simulink model "Luenb_no_integr_sim_model"  (R2020a)
settings: Solver=ode3  StartTime=0.0  StopTime=600  FixedStep=Ts  RelTol=1e-3  EnableMultiTasking=on
values from neighbouring files (symbols this model uses):
  A = Model.A    [GPB1_estimation.m]    (also in GPB1_estimation_BT.m; GPB2_estimation.m)
  B = Model.B    [GPB1_estimation_BT.m]
  C = Model.C    [GPB1_estimation.m]    (also in GPB1_estimation_BT.m; GPB2_estimation.m; MKFObserverA.m = obj.filters{f}.C)
  K = Pred_P * C{j}' / S    [GPB1_estimation.m]    (also in GPB1_estimation_BT.m; GPB2_estimation.m)
  x0 = zeros(n, 1)    [AbstractLinearFilter.m]    (also in KalmanFilter.m; KalmanFilterSS_sfunc.m = obs.xkp1_est; MEKF_observer_RODD.m; MKFObserver.m)
undefined symbols (not defined in the file or in its folder): Ts
settings Model: Creator=desbiens  LastModifiedBy=billtubbs
settings DataIOCC: LimitDataPoints=on  SaveFormat=Array  SignalLoggingSaveFormat=ModelDataLogs  ReturnWorkspaceOutputs=off
settings OptimizationCC: ExpressionDepthLimit=2147483647  InitFltsAndDblsToZero=on  LifeSpan=inf
settings DebuggingCC: UnderspecifiedInitializationDetection=Classic  MergeDetectMultiDrivingBlocksExec=none  SolverPrmCheckMsg=warning  FcnCallInpInsideContextMsg=warning  StateNameClashWarn=warning  SFUnexpectedBacktrackingDiag=warning  SFNoUnconditionalDefaultTransitionDiag=warning  SFExecutionAtInitializationDiag=none  ArithmeticOperatorsInVariantConditions=warning
settings HardwareCC: ProdBitPerPointer=32  ProdBitPerSizeT=32  ProdBitPerPtrDiffT=32  ProdLargestAtomicFloat=None  ProdIntDivRoundTo=Undefined  ProdEndianess=Unspecified  ProdWordSize=32  ProdHWDeviceType=32-bit Generic
settings ModelReferenceCC: PropagateSignalLabelsOutOfModel=off
settings SFSimCC: SimUseLocalCustomCode=off  CustomCodeUndefinedFunction=UseInterfaceOnly
settings RTWCC: RTWUseLocalCustomCode=off
settings CodeAppCC: StateflowObjectComments=on
settings GRTTargetCC: TargetLangStandard=C89/C90 (ANSI)  CombineOutputUpdateFcns=off  GRTInterface=on
settings ConfigComp: CovMetricSettings=dw  CovHtmlReporting=on  CovSaveCumulativeToWorkspaceVar=on  CovSaveSingleToWorkspaceVar=on  CovExternalEMLEnable=off

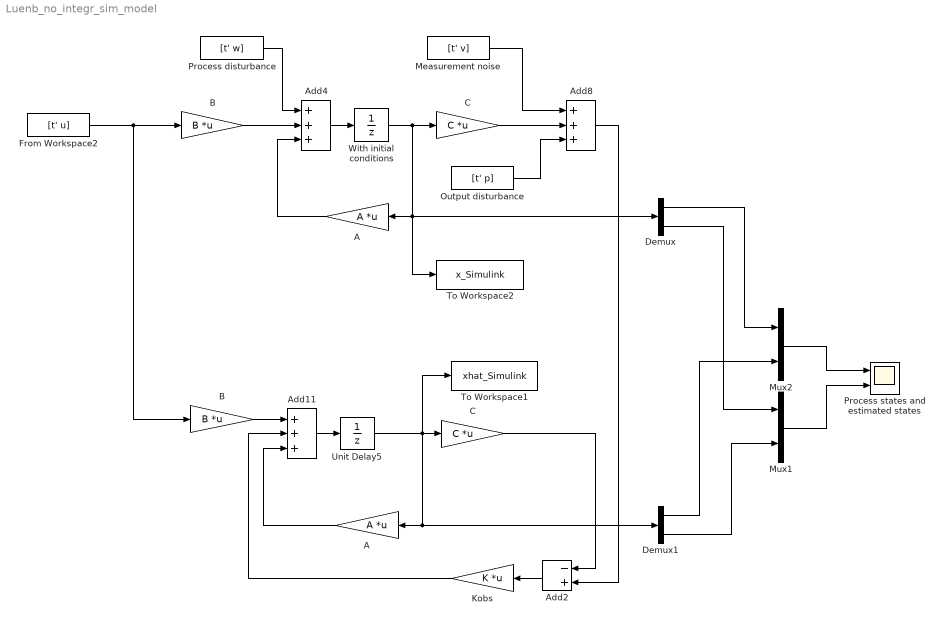
== system Luenb_no_integr_sim_model ==
  A : Gain  Gain=A  Multiplication=Matrix(K*u)
  "A " : Gain  Gain=A  Multiplication=Matrix(K*u)
  Add11 : Sum  Inputs=+++
  Add2 : Sum  Inputs=-+
  Add4 : Sum  Inputs=+++
  Add8 : Sum  Inputs=+++
  B : Gain  Gain=B  Multiplication=Matrix(K*u)
  "B " : Gain  Gain=B  Multiplication=Matrix(K*u)
  C : Gain  Gain=C  Multiplication=Matrix(K*u)
  "C " : Gain  Gain=C  Multiplication=Matrix(K*u)
  Demux : Demux  Outputs=2
  Demux1 : Demux  Outputs=2
  From Workspace2 : FromWorkspace  VariableName=[t' u]
  Kobs : Gain  Gain=K  Multiplication=Matrix(K*u)
  Measurement noise : FromWorkspace  VariableName=[t' v]
  Mux1 : Mux  Inputs=2
  Mux2 : Mux  Inputs=2
  Output disturbance : FromWorkspace  VariableName=[t' p]
  Process disturbance : FromWorkspace  VariableName=[t' w]
  Process states and estimated states : Scope  NumInputPorts=2
  To Workspace1 : ToWorkspace  VariableName=xhat_Simulink  SaveFormat=Timeseries  SampleTime=-1
  To Workspace2 : ToWorkspace  VariableName=x_Simulink  SaveFormat=Timeseries  SampleTime=-1
  Unit Delay5 : UnitDelay  SampleTime=Ts  HasFrameUpgradeWarning=on
  With initial conditions : UnitDelay  InitialCondition=x0  SampleTime=Ts  HasFrameUpgradeWarning=on
  wires:
  Measurement noise/1 -> Add8/1
  Add4/1 -> With initial conditions/1
  With initial conditions/1 -> C/1, To Workspace2/1, A/1, Demux/1
  C/1 -> Add8/2
  Add11/1 -> Unit Delay5/1
  "A "/1 -> Add11/3
  Unit Delay5/1 -> To Workspace1/1, "C "/1, "A "/1, Demux1/1
  Add8/1 -> Add2/2
  From Workspace2/1 -> "B "/1, B/1
  Output disturbance/1 -> Add8/3
  "B "/1 -> Add11/1
  Kobs/1 -> Add11/2
  Add2/1 -> Kobs/1
  "C "/1 -> Add2/1
  A/1 -> Add4/3
  B/1 -> Add4/2
  Process disturbance/1 -> Add4/1
  Mux1/1 -> Process states and estimated states/2
  Demux/2 -> Mux1/1
  Demux1/2 -> Mux1/2
  Demux/1 -> Mux2/1
  Mux2/1 -> Process states and estimated states/1
  Demux1/1 -> Mux2/2
